simulink model "VSG_2level"  (R2024b)
settings: Solver=ode23t  StartTime=0.0  StopTime=4  RelTol=1e-3
InitFcn:
  | Rf = 0.05;
  | fn = 50;
  | Ub = 380;
  | Sb = 150e3;
  | Ib = Sb/(sqrt(3)*Ub);
  | W0 = 2*pi*fn;
  | J = 3.36;
  | D = 3.24e4/W0;
  | Kf = 2.941e6/W0;
  | Kq = (9e4*Ub)/(Sb*sqrt(3));
  | Ki = 0.35*sqrt(3)*Sb/Ub;
  | L = 1e-3;
  | Cf = 35e-6;
  | R = 0.1;
  | Un = 380;
undefined symbols (not defined in the file or in its folder): Ion, Lithium
libraries: spsSeriesRLCBranchLib x13, spsIGBTDiodeLib x10, slpidlib x7, spsThreePhaseVIMeasurementLib x4, spsabctodq0Lib x4, spsVoltageMeasurementLib x4, spsPowerPositiveSequenceLib x3, simulink x3, spsBatteryLib x2, spsPLL3phLib x2, spsThreePhaseSeriesRLCLoadLib x2, spsThreePhaseBreakerLib x2
(part 1 of 2)
settings Model: Creator=ASUS  LastModifiedBy=ASUS
settings DataIOCC: ReturnWorkspaceOutputs=off

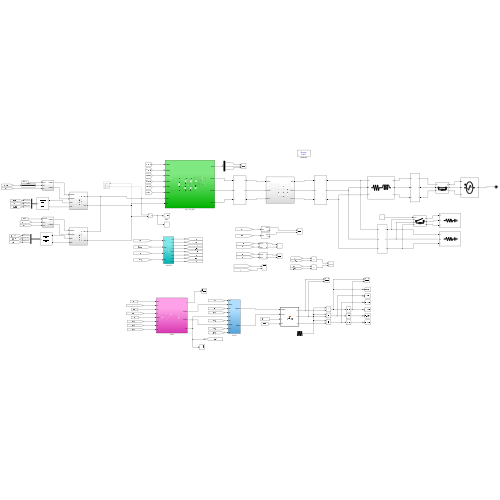
[thumbnail: Simulink's stored preview of the top-level diagram]
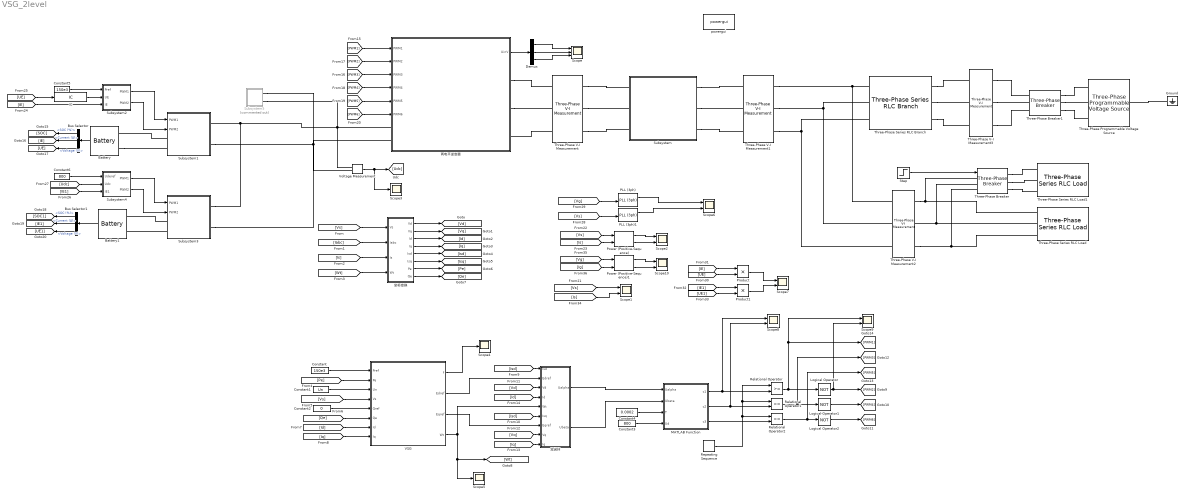
== system VSG_2level ==
  Battery : spsBatteryLib/Battery  BatType=Lithium-Ion  NomV=500  NomQ=100  SOC=80  Batt_Tr=30  PresetModel=on  MaxQ=100  MinV=375  FullV=581.9936  Dis_rate=43.4783  R=0.05  Normal_OP=90.4348  expZone="[540.1929      4.913043]"
  Battery1 : spsBatteryLib/Battery  BatType=Lithium-Ion  NomV=500  NomQ=50  SOC=80  Batt_Tr=30  PresetModel=on  MaxQ=50  MinV=375  FullV=581.9936  Dis_rate=21.7391  R=0.1  Normal_OP=45.2174  expZone="[540.1929      2.456522]"
  Bus Selector : BusSelector  OutputSignals=SOC (%),Current (A),Voltage (V)
  Bus Selector1 : BusSelector  OutputSignals=SOC (%),Current (A),Voltage (V)
  Constant : Constant  Value=150e3
  Constant1 : Constant  Value=Un
  Constant2 : Constant  Value=0
  Constant3 : Constant  Value=800
  Constant4 : Constant  Value=0.0002
  Constant5 : Constant  Value=150e3
  Constant6 : Constant  Value=800
  Demux : Demux  Outputs=3
  Ground : spsGroundLib/Ground  LConnTagsString=a
  IC : InitialCondition  Value=800
  Logical Operator : Logic  Operator=NOT  AllPortsSameDT=off  OutDataTypeStr=boolean
  Logical Operator1 : Logic  Operator=NOT  AllPortsSameDT=off  OutDataTypeStr=boolean
  Logical Operator2 : Logic  Operator=NOT  AllPortsSameDT=off  OutDataTypeStr=boolean
  MATLAB Function : MATLAB Function  TreatAsAtomicUnit=on
  PLL (3ph) : spsPLL3phLib/PLL (3ph)  Fmin=45  Par_Init=[0, 50]  ParK=[180, 3200, 1]  TcD=1e-4  MaxRateChangeFreq=12  FilterCutOffFreq=25  Ts=0  AGC=on
  PLL (3ph)1 : spsPLL3phLib/PLL (3ph)  Fmin=45  Par_Init=[0, 50]  ParK=[180, 3200, 1]  TcD=1e-4  MaxRateChangeFreq=12  FilterCutOffFreq=25  Ts=0  AGC=on
  Power (Positive-Sequence) : spsPowerPositiveSequenceLib/Power (Positive-Sequence)  Freq=60  Vinit=[0, 0]  Iinit=[0, 0]  Ts=0
      settings: LibrarySourceBlock=|
      | sps_lib/Sensors and Measurements/Power
      | (Positive-Sequence)
  Power (Positive-Sequence)1 : spsPowerPositiveSequenceLib/Power (Positive-Sequence)  Freq=60  Vinit=[0, 0]  Iinit=[0, 0]  Ts=0
      settings: LibrarySourceBlock=|
      | sps_lib/Sensors and Measurements/Power
      | (Positive-Sequence)
  Product : Product
  Product1 : Product
  Relational Operator : RelationalOperator  OutDataTypeStr=boolean  RndMeth=Simplest  InputSameDT=off
  Relational Operator1 : RelationalOperator  OutDataTypeStr=boolean  RndMeth=Simplest  InputSameDT=off
  Relational Operator2 : RelationalOperator  OutDataTypeStr=boolean  RndMeth=Simplest  InputSameDT=off
  Repeating Sequence : simulink/Sources/Repeating Sequence  rep_seq_t=[0 1/10000 0.0002]  rep_seq_y=[0 1/10000 0]
  Scope : Scope  NumInputPorts=3
  Scope{1..2,6..10} (7 alike) : Scope  NumInputPorts=2
  Scope3 : Scope
  Scope4 : Scope
  Scope5 : Scope
  Step : Step  SampleTime=0
  Subsystem : Subsystem
  Subsystem1 : Subsystem
  Subsystem2 : Subsystem
  Subsystem3 : Subsystem
  Subsystem4 : Subsystem
  Subsystem5 : Subsystem  Commented=on
  Three-Phase Programmable Voltage Source : spsThreePhaseProgrammableVoltageSourceLib/Three-Phase Programmable Voltage Source  PositiveSequence=[380 0 50]  VariationEntity=Frequency  VariationType=Table of time-amplitude pairs  VariationTypeAlt=Step  VariationStep=0  VariationRate=10  VariationMagnitude=0.3  VariationFrequency=2  VariationTiming=[0 0]  VariationPhaseA=off  Amplitudes=[1 0.8 1.2 1.0]  TimeValues=[0 0.1 0.15 0.2]  HarmonicGeneration=off  HarmonicA=[3 0.2 -25 0]  HarmonicB=[2 0.15 35 2]  Timing="[0.05  3]"  BusType=swing  Pref=0  Qref=0  Qmin=-inf  Qmax=inf
  Three-Phase Series RLC Branch : spsThreePhaseSeriesRLCBranchLib/Three-Phase Series RLC Branch  LConnTagsString=A|B|C  RConnTagsString=A|B|C  BranchType=RL  Resistance=0.06  Inductance=1.35e-3  Capacitance=1e-6  Measurements=None
  Three-Phase Series RLC Load : spsThreePhaseSeriesRLCLoadLib/Three-Phase Series RLC Load  LConnTagsString=A|B|C  Configuration=Y (grounded)  NominalVoltage=380  Vabc=[1e3 1e3 1e3]  Vabcp=[1e3 1e3 1e3]  NominalFrequency=50  UnbalancedPower=off  ActivePower=100e3  InductivePower=0  CapacitivePower=0  Pabc=[10e3 9e3 11e3]  QLabc=[100 90 110]  QCabc=[100 90 110]  Pabcp=[10e3 9e3 11e3]  QLabcp=[100 90 110]  QCabcp=[100 90 110]  Measurements=None  LoadType=constant Z
  Three-Phase Series RLC Load1 : spsThreePhaseSeriesRLCLoadLib/Three-Phase Series RLC Load  LConnTagsString=A|B|C  Configuration=Y (grounded)  NominalVoltage=380  Vabc=[1e3 1e3 1e3]  Vabcp=[1e3 1e3 1e3]  NominalFrequency=50  UnbalancedPower=off  ActivePower=50e3  InductivePower=0  CapacitivePower=0  Pabc=[10e3 9e3 11e3]  QLabc=[100 90 110]  QCabc=[100 90 110]  Pabcp=[10e3 9e3 11e3]  QLabcp=[100 90 110]  QCabcp=[100 90 110]  Measurements=None  LoadType=constant Z
  Three-Phase V-I Measurement : spsThreePhaseVIMeasurementLib/Three-Phase V-I Measurement  VoltageMeasurement=no  SetLabelV=off  LabelV=Vabc  Vpu=off  VpuLL=off  CurrentMeasurement=yes  SetLabelI=on  LabelI=Iabc  Ipu=off  Pbase=100e6  Vbase=500e3  OutputType=Complex  PhasorSimulation=off  PSBequivalent=0
  Three-Phase V-I Measurement1 : spsThreePhaseVIMeasurementLib/Three-Phase V-I Measurement  VoltageMeasurement=phase-to-ground  SetLabelV=on  LabelV=Vs  Vpu=off  VpuLL=off  CurrentMeasurement=yes  SetLabelI=on  LabelI=Is  Ipu=off  Pbase=100e6  Vbase=500e3  OutputType=Complex  PhasorSimulation=off  PSBequivalent=0
  Three-Phase V-I Measurement2 : spsThreePhaseVIMeasurementLib/Three-Phase V-I Measurement  VoltageMeasurement=phase-to-ground  SetLabelV=on  LabelV=VL  Vpu=off  VpuLL=off  CurrentMeasurement=yes  SetLabelI=on  LabelI=IL  Ipu=off  Pbase=100e6  Vbase=500e3  OutputType=Complex  PhasorSimulation=off  PSBequivalent=0
  Three-Phase V-I Measurement3 : spsThreePhaseVIMeasurementLib/Three-Phase V-I Measurement  VoltageMeasurement=phase-to-ground  SetLabelV=on  LabelV=Vg  Vpu=off  VpuLL=off  CurrentMeasurement=yes  SetLabelI=on  LabelI=Ig  Ipu=off  Pbase=100e6  Vbase=500e3  OutputType=Complex  PhasorSimulation=off  PSBequivalent=0
  Three-Phase Breaker : spsThreePhaseBreakerLib/Three-Phase Breaker  InitialState=open  SwitchA=on  SwitchB=on  SwitchC=on  SwitchTimes="[1  5/60]"  External=on  BreakerResistance=0.0000001  SnubberResistance=1e10  SnubberCapacitance=inf  Measurements=None
  Three-Phase Breaker1 : spsThreePhaseBreakerLib/Three-Phase Breaker  InitialState=closed  SwitchA=on  SwitchB=on  SwitchC=on  SwitchTimes=[2]  External=off  BreakerResistance=0.0000001  SnubberResistance=1e10  SnubberCapacitance=inf  Measurements=None
  VSG : Subsystem
  Voltage Measurement : spsVoltageMeasurementLib/Voltage Measurement  PhasorSimulation=off  OutputType=Complex  PSBequivalent=0
  powergui : sps_lib/powergui  Priority=1  SimulationMode=Discrete  SampleTime=1e-6  frequency=60  Iterations=50  frequencyindice=0  Pbase=100e6  ErrMax=1e-4  UnitsV=kV  UnitsW=MW  buscounter=0  FunctionMessages=off  echomessages=off  EnableUseOfTLC=off  CurrentSourceSwitches=off  DisableSnubberDevices=off  DisableRonSwitches=off  DisableVfSwitches=off  DisplayEquations=off  AutomaticDiscreteSolvers=off  SolverType=Tustin/Backward Euler (TBE)  Interpol=off  ExternalGateDelay=off  methode=off  Ts=100  x0status=blocks  SPID=on  SwTol=0  HookPort=off  NonlinearTolerance=1e-4  nMaxIteration=100  ContinueOnMaxIteration=off  RestoreLinks=warning  ResistiveCurrentMeasurement=off  Frange=[0:2:500]  Ylog=off  Xlog=on  ShowGrid=off  save=off  variable=ZData  structure=0  ZoomFFT=off  StartTime=0.0  cycles=1  DisplayStyle=1  fundamental=60  FreqAxis=off  MaxFrequency=1000  frequencyindicesteady=1  RmsSteady=1  display=off
  两电平逆变器 : Subsystem
  双闭环 : Subsystem
  坐标变换 : Subsystem
  wires:
  [Vs] -> 坐标变换/1(Vs)
  [Iabc] -> 坐标变换/2(Iabc)
  [Is] -> 坐标变换/3(Is)
  [Wt] -> 坐标变换/4(Wt)
  坐标变换/1(Vd) -> [Vd]
  坐标变换/2(Vq) -> [Vq]
  坐标变换/3(Id) -> [Id]
  坐标变换/4(Iq) -> [Iq]
  坐标变换/5(Isd) -> [Isd]
  坐标变换/6(Isq) -> [Isq]
  坐标变换/7(Pe) -> [Pe]
  坐标变换/8(Qe) -> [Qe]
  Constant/1 -> VSG/1(Pref)
  [Pe] -> VSG/2(Pe)
  Constant1/1 -> VSG/3(Un)
  [Vs] -> VSG/4(Vs)
  Constant2/1 -> VSG/5(Qref)
  [Qe] -> VSG/6(Qe)
  [Id] -> VSG/7(Id)
  [Iq] -> VSG/8(Iq)
  VSG/2(Edref) -> 双闭环/2(Edref)
  VSG/3(Eqref) -> 双闭环/7(Eqref)
  [Isd] -> 双闭环/1(Isd)
  [Isd] -> 双闭环/6(Isq)
  VSG/4(Wt) -> 双闭环/5(Wt), [Wt], Scope5/1
  [Vd] -> 双闭环/3(Vd)
  [Vq] -> 双闭环/8(Vq)
  [Iq] -> 双闭环/9(Iq)
  [Id] -> 双闭环/4(Id)
  双闭环/1(Ualpha) -> MATLAB Function/1(Ualpha)
  双闭环/2(Ubeta) -> MATLAB Function/2(Ubeta)
  Constant3/1 -> MATLAB Function/4(Ud)
  Constant4/1 -> MATLAB Function/3(T)
  Repeating Sequence/1 -> Relational Operator2/1, Relational Operator1/1, Relational Operator/1
  MATLAB Function/1(c1) -> Scope8/1, Relational Operator/2
  MATLAB Function/2(c2) -> Scope8/2, Relational Operator1/2
  MATLAB Function/3(c3) -> Relational Operator2/2
  Relational Operator/1 -> Scope9/1, [PWM1], Logical Operator/1
  Relational Operator1/1 -> [PWM3], Logical Operator1/1
  Relational Operator2/1 -> [PWM5], Logical Operator2/1
  Logical Operator/1 -> Scope9/2, [PWM2]
  Logical Operator1/1 -> [PWM4]
  Logical Operator2/1 -> [PWM6]
  [PWM6] -> 两电平逆变器/6(PWM6)
  [PWM5] -> 两电平逆变器/5(PWM5)
  [PWM4] -> 两电平逆变器/4(PWM4)
  [PWM3] -> 两电平逆变器/3(PWM3)
  [PWM2] -> 两电平逆变器/2(PWM2)
  [PWM1] -> 两电平逆变器/1(PWM1)
  两电平逆变器/1(UinV) -> Demux/1
  Demux/2 -> Scope/2
  Demux/1 -> Scope/1
  Demux/3 -> Scope/3
  [Vs] -> Scope1/1
  [Vs] -> Power (Positive-Sequence)/1
  [Is] -> Power (Positive-Sequence)/2
  Power (Positive-Sequence)/1 -> Scope2/1
  Power (Positive-Sequence)/2 -> Scope2/2
  Battery/1 -> Bus Selector/1
  Bus Selector/1 -> [SOC]  "<SOC (%)>"
  Bus Selector/2 -> [IE]  "<Current (A)>"
  Bus Selector/3 -> [UE]  "<Voltage (V)>"
  [UE] -> IC/1
  [IE] -> Subsystem2/3(IE)
  Constant5/1 -> Subsystem2/1(Pref)
  Subsystem2/1(PWM1) -> Subsystem1/1(PWM1)
  Subsystem2/2(PWM2) -> Subsystem1/2(PWM2)
  Subsystem4/2(PWM2) -> Subsystem3/2(PWM2)
  Subsystem4/1(PWM1) -> Subsystem3/1(PWM1)
  Constant6/1 -> Subsystem4/1(Uderef)
  [IE1] -> Subsystem4/3(IE1)
  [Udc] -> Subsystem4/2(Udc)
  Bus Selector1/3 -> [UE1]  "<Voltage (V)>"
  Bus Selector1/2 -> [IE1]  "<Current (A)>"
  Bus Selector1/1 -> [SOC1]  "<SOC (%)>"
  Battery1/1 -> Bus Selector1/1
  Voltage Measurement/1 -> Scope3/1, [Udc]
  IC/1 -> Subsystem2/2(UE)
  VSG/1(f) -> Scope4/1
  [Vg] -> PLL (3ph)/1
  [Vs] -> PLL (3ph)1/1
  PLL (3ph)/1 -> Scope6/1
  PLL (3ph)1/1 -> Scope6/2
  [IE] -> Product/1
  [UE] -> Product/2
  [UE1] -> Product1/2
  [IE1] -> Product1/1
  Product/1 -> Scope7/1
  Product1/1 -> Scope7/2
  [Is] -> Scope1/2
  Power (Positive-Sequence)1/2 -> Scope10/2
  Power (Positive-Sequence)1/1 -> Scope10/1
  [Ig] -> Power (Positive-Sequence)1/2
  [Vg] -> Power (Positive-Sequence)1/1
  Step/1 -> Three-Phase Breaker/1
  connections:
  两电平逆变器/RConn1 -- Three-Phase V-I Measurement/LConn1
  两电平逆变器/RConn2 -- Three-Phase V-I Measurement/LConn2
  Three-Phase V-I Measurement/LConn3 -- 两电平逆变器/RConn3
  Three-Phase V-I Measurement/RConn1 -- Subsystem/LConn1
  Three-Phase V-I Measurement/RConn2 -- Subsystem/LConn2
  Three-Phase V-I Measurement/RConn3 -- Subsystem/LConn3
  Subsystem/RConn1 -- Three-Phase V-I Measurement1/LConn1
  Subsystem/RConn2 -- Three-Phase V-I Measurement1/LConn2
  Subsystem/RConn3 -- Three-Phase V-I Measurement1/LConn3
  Three-Phase V-I Measurement2/RConn1 -- Three-Phase Breaker/LConn1 -- Three-Phase Series RLC Load/LConn1
  Three-Phase Series RLC Load/LConn2 -- Three-Phase Breaker/LConn2 -- Three-Phase V-I Measurement2/RConn2
  Three-Phase V-I Measurement2/RConn3 -- Three-Phase Breaker/LConn3 -- Three-Phase Series RLC Load/LConn3
  Three-Phase V-I Measurement1/RConn1 -- Three-Phase Series RLC Branch/LConn1 -- Three-Phase V-I Measurement2/LConn1
  Three-Phase V-I Measurement1/RConn2 -- Three-Phase Series RLC Branch/LConn2 -- Three-Phase V-I Measurement2/LConn2
  Three-Phase V-I Measurement1/RConn3 -- Three-Phase Series RLC Branch/LConn3 -- Three-Phase V-I Measurement2/LConn3
  Three-Phase Series RLC Branch/RConn1 -- Three-Phase V-I Measurement3/LConn1
  Three-Phase Series RLC Branch/RConn2 -- Three-Phase V-I Measurement3/LConn2
  Three-Phase Series RLC Branch/RConn3 -- Three-Phase V-I Measurement3/LConn3
  Ground/LConn1 -- Three-Phase Programmable Voltage Source/LConn1
  Battery/LConn2 -- Subsystem1/LConn2
  Subsystem3/LConn2 -- Battery1/LConn2
  Subsystem3/LConn1 -- Battery1/LConn1
  两电平逆变器/LConn1 -- Subsystem3/RConn1 -- Subsystem1/RConn1 -- Subsystem5/LConn2 -- Voltage Measurement/LConn1
  Subsystem1/RConn2 -- Subsystem5/LConn1 -- 两电平逆变器/LConn2 -- Subsystem3/RConn2 -- Voltage Measurement/LConn2
  Subsystem1/LConn1 -- Battery/LConn1
  Three-Phase Breaker/RConn2 -- Three-Phase Series RLC Load1/LConn2
  Three-Phase Breaker/RConn3 -- Three-Phase Series RLC Load1/LConn3
  Three-Phase V-I Measurement3/RConn1 -- Three-Phase Breaker1/LConn1
  Three-Phase V-I Measurement3/RConn2 -- Three-Phase Breaker1/LConn2
  Three-Phase V-I Measurement3/RConn3 -- Three-Phase Breaker1/LConn3
  Three-Phase Breaker1/RConn2 -- Three-Phase Programmable Voltage Source/RConn2
  Three-Phase Breaker1/RConn1 -- Three-Phase Programmable Voltage Source/RConn1
  Three-Phase Breaker1/RConn3 -- Three-Phase Programmable Voltage Source/RConn3
  Three-Phase Breaker/RConn1 -- Three-Phase Series RLC Load1/LConn1

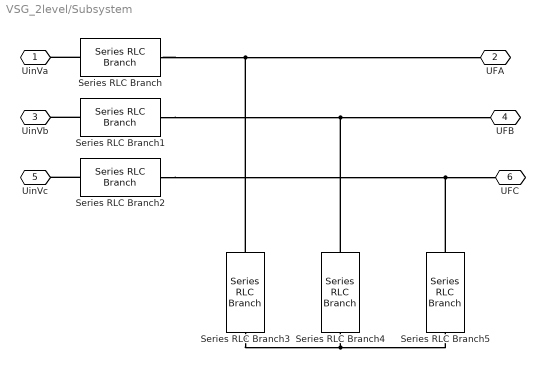
== system VSG_2level/Subsystem ==
  Series RLC Branch : spsSeriesRLCBranchLib/Series RLC Branch  LConnTagsString=__new0  RConnTagsString=__new0  BranchType=RL  Resistance=Rf  Inductance=L  SetiL0=off  InitialCurrent=0  Capacitance=1e-6  Setx0=off  InitialVoltage=0  Measurements=None
  Series RLC Branch1 : spsSeriesRLCBranchLib/Series RLC Branch  LConnTagsString=__new0  RConnTagsString=__new0  BranchType=RL  Resistance=Rf  Inductance=L  SetiL0=off  InitialCurrent=0  Capacitance=1e-6  Setx0=off  InitialVoltage=0  Measurements=None
  Series RLC Branch2 : spsSeriesRLCBranchLib/Series RLC Branch  LConnTagsString=__new0  RConnTagsString=__new0  BranchType=RL  Resistance=Rf  Inductance=L  SetiL0=off  InitialCurrent=0  Capacitance=1e-6  Setx0=off  InitialVoltage=0  Measurements=None
  Series RLC Branch3 : spsSeriesRLCBranchLib/Series RLC Branch  LConnTagsString=__new0  RConnTagsString=__new0  BranchType=RC  Resistance=Rf  Inductance=L  SetiL0=off  InitialCurrent=0  Capacitance=Cf  Setx0=off  InitialVoltage=0  Measurements=None
  Series RLC Branch4 : spsSeriesRLCBranchLib/Series RLC Branch  LConnTagsString=__new0  RConnTagsString=__new0  BranchType=RC  Resistance=Rf  Inductance=L  SetiL0=off  InitialCurrent=0  Capacitance=Cf  Setx0=off  InitialVoltage=0  Measurements=None
  Series RLC Branch5 : spsSeriesRLCBranchLib/Series RLC Branch  LConnTagsString=__new0  RConnTagsString=__new0  BranchType=RC  Resistance=Rf  Inductance=L  SetiL0=off  InitialCurrent=0  Capacitance=Cf  Setx0=off  InitialVoltage=0  Measurements=None
  UinVa : PMIOPort  Side=Left
  UFA : PMIOPort  Port=2  Side=Right
  UinVb : PMIOPort  Port=3  Side=Left
  UFB : PMIOPort  Port=4  Side=Right
  UinVc : PMIOPort  Port=5  Side=Left
  UFC : PMIOPort  Port=6  Side=Right
  connections:
  Series RLC Branch3/RConn1 -- Series RLC Branch5/RConn1 -- Series RLC Branch4/RConn1
  Series RLC Branch/RConn1 -- UFA/RConn1 -- Series RLC Branch3/LConn1
  Series RLC Branch2/RConn1 -- UFC/RConn1 -- Series RLC Branch5/LConn1
  Series RLC Branch1/RConn1 -- UFB/RConn1 -- Series RLC Branch4/LConn1
  Series RLC Branch1/LConn1 -- UinVb/RConn1
  Series RLC Branch/LConn1 -- UinVa/RConn1
  Series RLC Branch2/LConn1 -- UinVc/RConn1

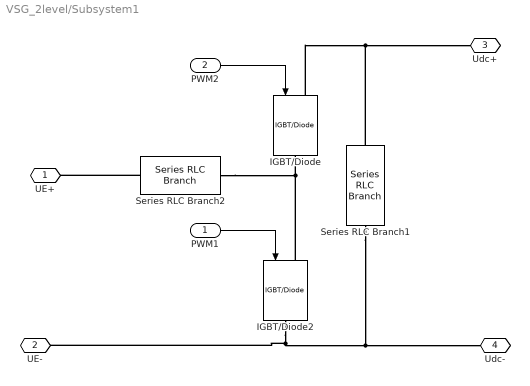
== system VSG_2level/Subsystem1 ==
  PWM1 : Inport
  PWM2 : Inport  Port=2
  IGBT/Diode : spsIGBTDiodeLib/IGBT//Diode  Ron=1e-3  Rs=1e5  Cs=inf  Measurements=off
  IGBT/Diode2 : spsIGBTDiodeLib/IGBT//Diode  Ron=1e-3  Rs=1e5  Cs=inf  Measurements=off
  Series RLC Branch1 : spsSeriesRLCBranchLib/Series RLC Branch  LConnTagsString=__new0  RConnTagsString=__new0  BranchType=C  Resistance=1  Inductance=1.68e-3  SetiL0=off  InitialCurrent=0  Capacitance=5.5e-3  Setx0=on  InitialVoltage=800  Measurements=None
  Series RLC Branch2 : spsSeriesRLCBranchLib/Series RLC Branch  LConnTagsString=__new0  RConnTagsString=__new0  BranchType=L  Resistance=1  Inductance=1.68e-3  SetiL0=off  InitialCurrent=0  Capacitance=1e-6  Setx0=off  InitialVoltage=0  Measurements=None
  UE+ : PMIOPort  Side=Left
  UE- : PMIOPort  Port=2  Side=Left
  Udc+ : PMIOPort  Port=3  Side=Right
  Udc- : PMIOPort  Port=4  Side=Right
  wires:
  PWM1/1 -> IGBT/Diode2/1
  PWM2/1 -> IGBT/Diode/1
  connections:
  Series RLC Branch2/LConn1 -- UE+/RConn1
  IGBT/Diode2/LConn1 -- IGBT/Diode/RConn1 -- Series RLC Branch2/RConn1
  IGBT/Diode/LConn1 -- Udc+/RConn1 -- Series RLC Branch1/LConn1
  IGBT/Diode2/RConn1 -- UE-/RConn1 -- Udc-/RConn1 -- Series RLC Branch1/RConn1

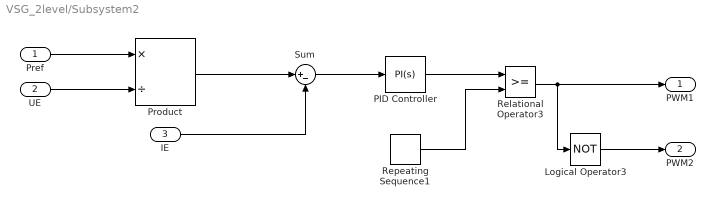
== system VSG_2level/Subsystem2 ==
  Pref : Inport
  UE : Inport  Port=2
  IE : Inport  Port=3
  Logical Operator3 : Logic  Operator=NOT  AllPortsSameDT=off  OutDataTypeStr=boolean
  PID Controller : slpidlib/PID Controller  Controller=PI  Form=Parallel  TimeDomain=Continuous-time  UseExternalTs=off  SampleTime=-1  IntegratorMethod=Forward Euler  FilterMethod=Forward Euler  ControllerParametersSource=internal  P=0.715  I=1.12  UseKiTs=off  D=0  UseExternalDerivativeSource=off  N=100  UseFilter=on  TunerSelectOption=Transfer Function Based (PID Tuner App)  InitialConditionSource=internal  InitialConditionForIntegrator=0  InitialConditionForFilter=0  DifferentiatorICPrevScaledInput=0  ExternalReset=none  TrackingMode=off  Kt=1  LimitOutput=off  SatLimitsSource=internal  UpperSaturationLimit=1e10  LowerSaturationLimit=-1e10  LinearizeAsGain=on  AntiWindupMode=none  Kb=1  LimitIntegrator=off  UpperIntegratorSaturationLimit=1e10  LowerIntegratorSaturationLimit=-1e10  POutMin=[]  POutMax=[]  IOutMin=[]  IOutMax=[]  DOutMin=[]  DOutMax=[]  NOutMin=[]  NOutMax=[]  SumOutMin=[]  SumOutMax=[]  SaturationOutMin=[]  SaturationOutMax=[]  PParamMin=[]  PParamMax=[]  IParamMin=[]  IParamMax=[]  DParamMin=[]  DParamMax=[]  NParamMin=[]  NParamMax=[]  KbParamMin=[]  KbParamMax=[]  KtParamMin=[]  KtParamMax=[]  KbOutMin=[]  KbOutMax=[]  KtOutMin=[]  KtOutMax=[]  IntegratorOutMin=[]  IntegratorOutMax=[]  FilterOutMin=[]  FilterOutMax=[]  SumI1OutMin=[]  SumI1OutMax=[]  SumI2OutMin=[]  SumI2OutMax=[]  SumI3OutMin=[]  SumI3OutMax=[]  SumI4OutMin=[]  SumI4OutMax=[]  SumDOutMin=[]  SumDOutMax=[]  DifferentiatorOutMin=[]  DifferentiatorOutMax=[]  FilterDiffOutCoefMin=[]  FilterDiffOutCoefMax=[]  ReciprocalOutMin=[]  ReciprocalOutMax=[]  SumDenOutMin=[]  SumDenOutMax=[]  SumNumOutMin=[]  SumNumOutMax=[]  DivideOutMin=[]  DivideOutMax=[]  UdiffTsProdOutMin=[]  UdiffTsProdOutMax=[]  NTsProdOutMin=[]  NTsProdOutMax=[]  UintegralTsProdOutMin=[]  UintegralTsProdOutMax=[]  UngainTsProdOutMin=[]  UngainTsProdOutMax=[]  ClampingZeroOutDataTypeStr=Inherit: Inherit via back propagation  ClampingZeroOutMin=[]  ClampingZeroOutMax=[]  FilterDenConstantOutDataTypeStr=Inherit: Inherit via back propagation  FilterDenConstantOutMin=[]  FilterDenConstantOutMax=[]  PCopyOutDataTypeStr=Inherit: Inherit via back propagation  PCopyOutMin=[]  PCopyOutMax=[]  NCopyOutDataTypeStr=Inherit: Inherit via back propagation  NCopyOutMin=[]  NCopyOutMax=[]  IntegratorContinuousStateAttributes=''  IntegratorStateMustResolveToSignalObject=off  IntegratorRTWStateStorageClass=Auto  FilterContinuousStateAttributes=''  FilterStateMustResolveToSignalObject=off  FilterRTWStateStorageClass=Auto  ParallelPVariant=InternalParameters  IdealPVariant=Disabled  IVariant=InternalParameters  DVariant=Disabled  IntegratorVariant=Continuous  SatVariant=Disabled  AWVariant=Passthrough  PCopyVariant=Disabled  TRVariant=Disabled  FdbkBlocksVariant=Forward  IdealPFdbkVariant=Disabled  SatFdbkVariant=Disabled  DerivativeFilterVariant=Disabled  NVariant=Disabled  NCopyVariant=Disabled_SignalSpec  FilterICVariant=Disabled  IntegratorICVariant=InternalICs  ExternalResetVariant=Disabled  TRSumVariant=Passthrough  SumFdbkVariant=Disabled  SumVariant=Sum_PI  TsampFilterVariant=InternalTs  TsampNgainVariant=Passthrough  TsampIntegralVariant=Disabled_SignalSpec  ExternalSaturationOutDataTypeStr=Inherit: Same as second input  DerivativeSourceVariant=Disabled  PreIntVariant=InternalPreInt
  Product : Product  Inputs=*/
  Relational Operator3 : RelationalOperator  OutDataTypeStr=boolean  RndMeth=Simplest  InputSameDT=off
  Repeating Sequence1 : simulink/Sources/Repeating Sequence  rep_seq_t=[0 0.0001]  rep_seq_y=[0 1]
  Sum : Sum  Inputs=|+-
  PWM1 : Outport
  PWM2 : Outport  Port=2
  wires:
  Sum/1 -> PID Controller/1
  Product/1 -> Sum/1
  Pref/1 -> Product/1
  UE/1 -> Product/2
  IE/1 -> Sum/2
  Logical Operator3/1 -> PWM2/1
  Relational Operator3/1 -> PWM1/1, Logical Operator3/1
  Repeating Sequence1/1 -> Relational Operator3/2
  PID Controller/1 -> Relational Operator3/1

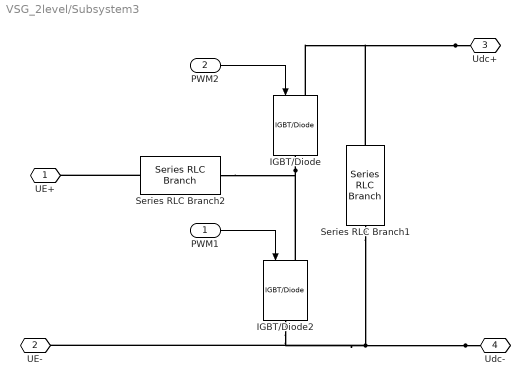
== system VSG_2level/Subsystem3 ==
  PWM1 : Inport
  PWM2 : Inport  Port=2
  IGBT/Diode : spsIGBTDiodeLib/IGBT//Diode  Ron=1e-3  Rs=1e5  Cs=inf  Measurements=off
  IGBT/Diode2 : spsIGBTDiodeLib/IGBT//Diode  Ron=1e-3  Rs=1e5  Cs=inf  Measurements=off
  Series RLC Branch1 : spsSeriesRLCBranchLib/Series RLC Branch  LConnTagsString=__new0  RConnTagsString=__new0  BranchType=C  Resistance=1  Inductance=1.68e-3  SetiL0=off  InitialCurrent=0  Capacitance=5.5e-3  Setx0=on  InitialVoltage=800  Measurements=None
  Series RLC Branch2 : spsSeriesRLCBranchLib/Series RLC Branch  LConnTagsString=__new0  RConnTagsString=__new0  BranchType=L  Resistance=1  Inductance=1.68e-3  SetiL0=off  InitialCurrent=0  Capacitance=1e-6  Setx0=off  InitialVoltage=0  Measurements=None
  UE+ : PMIOPort  Side=Left
  UE- : PMIOPort  Port=2  Side=Left
  Udc+ : PMIOPort  Port=3  Side=Right
  Udc- : PMIOPort  Port=4  Side=Right
  wires:
  PWM2/1 -> IGBT/Diode/1
  PWM1/1 -> IGBT/Diode2/1
  connections:
  Udc-/RConn1 -- IGBT/Diode2/RConn1 -- UE-/RConn1 -- Series RLC Branch1/RConn1
  Udc+/RConn1 -- IGBT/Diode/LConn1 -- Series RLC Branch1/LConn1
  IGBT/Diode/RConn1 -- Series RLC Branch2/RConn1 -- IGBT/Diode2/LConn1
  Series RLC Branch2/LConn1 -- UE+/RConn1

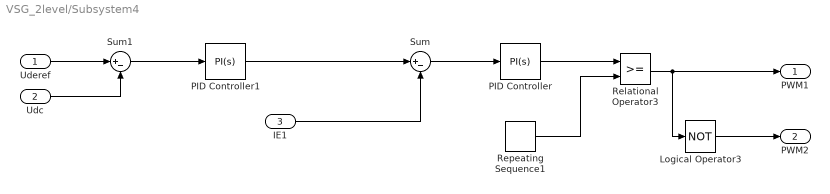
== system VSG_2level/Subsystem4 ==
  Uderef : Inport
  Udc : Inport  Port=2
  IE1 : Inport  Port=3
  Logical Operator3 : Logic  Operator=NOT  AllPortsSameDT=off  OutDataTypeStr=boolean
  PID Controller : slpidlib/PID Controller  Controller=PI  Form=Parallel  TimeDomain=Continuous-time  UseExternalTs=off  SampleTime=-1  IntegratorMethod=Forward Euler  FilterMethod=Forward Euler  ControllerParametersSource=internal  P=2.75  I=3.12  UseKiTs=off  D=0  UseExternalDerivativeSource=off  N=100  UseFilter=on  TunerSelectOption=Transfer Function Based (PID Tuner App)  InitialConditionSource=internal  InitialConditionForIntegrator=0  InitialConditionForFilter=0  DifferentiatorICPrevScaledInput=0  ExternalReset=none  TrackingMode=off  Kt=1  LimitOutput=off  SatLimitsSource=internal  UpperSaturationLimit=inf  LowerSaturationLimit=-inf  LinearizeAsGain=on  AntiWindupMode=none  Kb=1  LimitIntegrator=off  UpperIntegratorSaturationLimit=inf  LowerIntegratorSaturationLimit=-inf  POutMin=[]  POutMax=[]  IOutMin=[]  IOutMax=[]  DOutMin=[]  DOutMax=[]  NOutMin=[]  NOutMax=[]  SumOutMin=[]  SumOutMax=[]  SaturationOutMin=[]  SaturationOutMax=[]  PParamMin=[]  PParamMax=[]  IParamMin=[]  IParamMax=[]  DParamMin=[]  DParamMax=[]  NParamMin=[]  NParamMax=[]  KbParamMin=[]  KbParamMax=[]  KtParamMin=[]  KtParamMax=[]  KbOutMin=[]  KbOutMax=[]  KtOutMin=[]  KtOutMax=[]  IntegratorOutMin=[]  IntegratorOutMax=[]  FilterOutMin=[]  FilterOutMax=[]  SumI1OutMin=[]  SumI1OutMax=[]  SumI2OutMin=[]  SumI2OutMax=[]  SumI3OutMin=[]  SumI3OutMax=[]  SumI4OutMin=[]  SumI4OutMax=[]  SumDOutMin=[]  SumDOutMax=[]  DifferentiatorOutMin=[]  DifferentiatorOutMax=[]  FilterDiffOutCoefMin=[]  FilterDiffOutCoefMax=[]  ReciprocalOutMin=[]  ReciprocalOutMax=[]  SumDenOutMin=[]  SumDenOutMax=[]  SumNumOutMin=[]  SumNumOutMax=[]  DivideOutMin=[]  DivideOutMax=[]  UdiffTsProdOutMin=[]  UdiffTsProdOutMax=[]  NTsProdOutMin=[]  NTsProdOutMax=[]  UintegralTsProdOutMin=[]  UintegralTsProdOutMax=[]  UngainTsProdOutMin=[]  UngainTsProdOutMax=[]  ClampingZeroOutDataTypeStr=Inherit: Inherit via back propagation  ClampingZeroOutMin=[]  ClampingZeroOutMax=[]  FilterDenConstantOutDataTypeStr=Inherit: Inherit via back propagation  FilterDenConstantOutMin=[]  FilterDenConstantOutMax=[]  PCopyOutDataTypeStr=Inherit: Inherit via back propagation  PCopyOutMin=[]  PCopyOutMax=[]  NCopyOutDataTypeStr=Inherit: Inherit via back propagation  NCopyOutMin=[]  NCopyOutMax=[]  IntegratorContinuousStateAttributes=''  IntegratorStateMustResolveToSignalObject=off  IntegratorRTWStateStorageClass=Auto  FilterContinuousStateAttributes=''  FilterStateMustResolveToSignalObject=off  FilterRTWStateStorageClass=Auto  ParallelPVariant=InternalParameters  IdealPVariant=Disabled  IVariant=InternalParameters  DVariant=Disabled  IntegratorVariant=Continuous  SatVariant=Disabled  AWVariant=Passthrough  PCopyVariant=Disabled  TRVariant=Disabled  FdbkBlocksVariant=Forward  IdealPFdbkVariant=Disabled  SatFdbkVariant=Disabled  DerivativeFilterVariant=Disabled  NVariant=Disabled  NCopyVariant=Disabled_SignalSpec  FilterICVariant=Disabled  IntegratorICVariant=InternalICs  ExternalResetVariant=Disabled  TRSumVariant=Passthrough  SumFdbkVariant=Disabled  SumVariant=Sum_PI  TsampFilterVariant=InternalTs  TsampNgainVariant=Passthrough  TsampIntegralVariant=Disabled_SignalSpec  ExternalSaturationOutDataTypeStr=Inherit: Same as second input  DerivativeSourceVariant=Disabled  PreIntVariant=InternalPreInt
  PID Controller1 : slpidlib/PID Controller  Controller=PI  Form=Parallel  TimeDomain=Continuous-time  UseExternalTs=off  SampleTime=-1  IntegratorMethod=Forward Euler  FilterMethod=Forward Euler  ControllerParametersSource=internal  P=25  I=10.12  UseKiTs=off  D=0  UseExternalDerivativeSource=off  N=100  UseFilter=on  TunerSelectOption=Transfer Function Based (PID Tuner App)  InitialConditionSource=internal  InitialConditionForIntegrator=0  InitialConditionForFilter=0  DifferentiatorICPrevScaledInput=0  ExternalReset=none  TrackingMode=off  Kt=1  LimitOutput=off  SatLimitsSource=internal  UpperSaturationLimit=inf  LowerSaturationLimit=-inf  LinearizeAsGain=on  AntiWindupMode=none  Kb=1  LimitIntegrator=off  UpperIntegratorSaturationLimit=inf  LowerIntegratorSaturationLimit=-inf  POutMin=[]  POutMax=[]  IOutMin=[]  IOutMax=[]  DOutMin=[]  DOutMax=[]  NOutMin=[]  NOutMax=[]  SumOutMin=[]  SumOutMax=[]  SaturationOutMin=[]  SaturationOutMax=[]  PParamMin=[]  PParamMax=[]  IParamMin=[]  IParamMax=[]  DParamMin=[]  DParamMax=[]  NParamMin=[]  NParamMax=[]  KbParamMin=[]  KbParamMax=[]  KtParamMin=[]  KtParamMax=[]  KbOutMin=[]  KbOutMax=[]  KtOutMin=[]  KtOutMax=[]  IntegratorOutMin=[]  IntegratorOutMax=[]  FilterOutMin=[]  FilterOutMax=[]  SumI1OutMin=[]  SumI1OutMax=[]  SumI2OutMin=[]  SumI2OutMax=[]  SumI3OutMin=[]  SumI3OutMax=[]  SumI4OutMin=[]  SumI4OutMax=[]  SumDOutMin=[]  SumDOutMax=[]  DifferentiatorOutMin=[]  DifferentiatorOutMax=[]  FilterDiffOutCoefMin=[]  FilterDiffOutCoefMax=[]  ReciprocalOutMin=[]  ReciprocalOutMax=[]  SumDenOutMin=[]  SumDenOutMax=[]  SumNumOutMin=[]  SumNumOutMax=[]  DivideOutMin=[]  DivideOutMax=[]  UdiffTsProdOutMin=[]  UdiffTsProdOutMax=[]  NTsProdOutMin=[]  NTsProdOutMax=[]  UintegralTsProdOutMin=[]  UintegralTsProdOutMax=[]  UngainTsProdOutMin=[]  UngainTsProdOutMax=[]  ClampingZeroOutDataTypeStr=Inherit: Inherit via back propagation  ClampingZeroOutMin=[]  ClampingZeroOutMax=[]  FilterDenConstantOutDataTypeStr=Inherit: Inherit via back propagation  FilterDenConstantOutMin=[]  FilterDenConstantOutMax=[]  PCopyOutDataTypeStr=Inherit: Inherit via back propagation  PCopyOutMin=[]  PCopyOutMax=[]  NCopyOutDataTypeStr=Inherit: Inherit via back propagation  NCopyOutMin=[]  NCopyOutMax=[]  IntegratorContinuousStateAttributes=''  IntegratorStateMustResolveToSignalObject=off  IntegratorRTWStateStorageClass=Auto  FilterContinuousStateAttributes=''  FilterStateMustResolveToSignalObject=off  FilterRTWStateStorageClass=Auto  ParallelPVariant=InternalParameters  IdealPVariant=Disabled  IVariant=InternalParameters  DVariant=Disabled  IntegratorVariant=Continuous  SatVariant=Disabled  AWVariant=Passthrough  PCopyVariant=Disabled  TRVariant=Disabled  FdbkBlocksVariant=Forward  IdealPFdbkVariant=Disabled  SatFdbkVariant=Disabled  DerivativeFilterVariant=Disabled  NVariant=Disabled  NCopyVariant=Disabled_SignalSpec  FilterICVariant=Disabled  IntegratorICVariant=InternalICs  ExternalResetVariant=Disabled  TRSumVariant=Passthrough  SumFdbkVariant=Disabled  SumVariant=Sum_PI  TsampFilterVariant=InternalTs  TsampNgainVariant=Passthrough  TsampIntegralVariant=Disabled_SignalSpec  ExternalSaturationOutDataTypeStr=Inherit: Same as second input  DerivativeSourceVariant=Disabled  PreIntVariant=InternalPreInt
  Relational Operator3 : RelationalOperator  OutDataTypeStr=boolean  RndMeth=Simplest  InputSameDT=off
  Repeating Sequence1 : simulink/Sources/Repeating Sequence  rep_seq_t=[0 0.0001]  rep_seq_y=[0 1]
  Sum : Sum  Inputs=|+-
  Sum1 : Sum  Inputs=|+-
  PWM1 : Outport
  PWM2 : Outport  Port=2
  wires:
  PID Controller/1 -> Relational Operator3/1
  Repeating Sequence1/1 -> Relational Operator3/2
  Relational Operator3/1 -> Logical Operator3/1, PWM1/1
  Logical Operator3/1 -> PWM2/1
  IE1/1 -> Sum/2
  PID Controller1/1 -> Sum/1
  Sum/1 -> PID Controller/1
  Uderef/1 -> Sum1/1
  Udc/1 -> Sum1/2
  Sum1/1 -> PID Controller1/1

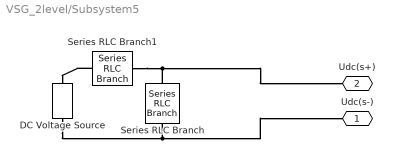
== system VSG_2level/Subsystem5 ==
  DC Voltage Source : spsDCVoltageSourceLib/DC Voltage Source  Amplitude=800  Measurements=None
  Series RLC Branch : spsSeriesRLCBranchLib/Series RLC Branch  LConnTagsString=__new0  RConnTagsString=__new0  BranchType=C  Resistance=1  Inductance=1e-3  SetiL0=off  InitialCurrent=0  Capacitance=1000e-6  Setx0=off  InitialVoltage=0  Measurements=None
  Series RLC Branch1 : spsSeriesRLCBranchLib/Series RLC Branch  LConnTagsString=__new0  RConnTagsString=__new0  BranchType=R  Resistance=0.000000000001  Inductance=1e-3  SetiL0=off  InitialCurrent=0  Capacitance=1000e-6  Setx0=off  InitialVoltage=0  Measurements=None
  Udc(s-) : PMIOPort  Side=Left
  Udc(s+) : PMIOPort  Port=2  Side=Left
  connections:
  Series RLC Branch1/LConn1 -- DC Voltage Source/RConn1
  Series RLC Branch/RConn1 -- Udc(s-)/RConn1 -- DC Voltage Source/LConn1
  Series RLC Branch1/RConn1 -- Udc(s+)/RConn1 -- Series RLC Branch/LConn1

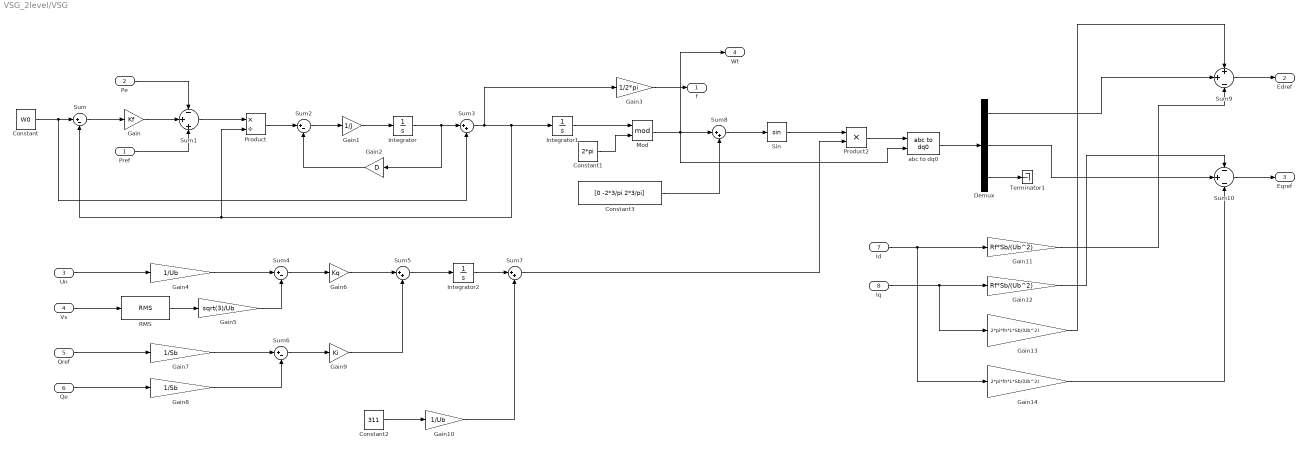
== system VSG_2level/VSG ==
  Pref : Inport
  Pe : Inport  Port=2
  Un : Inport  Port=3
  Vs : Inport  Port=4
  Qref : Inport  Port=5
  Qe : Inport  Port=6
  Id : Inport  Port=7
  Iq : Inport  Port=8
  Constant : Constant  Value=W0
  Constant1 : Constant  Value=2*pi
  Constant2 : Constant  Value=311
  Constant3 : Constant  Value=[0 -2*3/pi 2*3/pi]
  Demux : Demux  Outputs=3
  Gain : Gain  Gain=Kf
  Gain1 : Gain  Gain=1/J
  Gain10 : Gain  Gain=1/Ub
  Gain11 : Gain  Gain=Rf*Sb/(Ub^2)
  Gain12 : Gain  Gain=Rf*Sb/(Ub^2)
  Gain13 : Gain  Gain=2*pi*fn*L*Sb/(Ub^2)
  Gain14 : Gain  Gain=2*pi*fn*L*Sb/(Ub^2)
  Gain2 : Gain  Gain=D
  Gain3 : Gain  Gain=1/2*pi
  Gain4 : Gain  Gain=1/Ub
  Gain5 : Gain  Gain=sqrt(3)/Ub
  Gain6 : Gain  Gain=Kq
  Gain7 : Gain  Gain=1/Sb
  Gain8 : Gain  Gain=1/Sb
  Gain9 : Gain  Gain=Ki
  Integrator : Integrator  UpperSaturationLimit=100  LowerSaturationLimit=-100
  Integrator1 : Integrator
  Integrator2 : Integrator
  Mod : Math  Operator=mod
  Product : Product  Inputs=*/
  Product2 : Product
  RMS : dspstat3/RMS  run=off  directionMode=Each column  dimension=1  InputProcessing=Columns as channels (frame based)  reset_popup=None
  Sin : Trigonometry
  Sum{,2,4,6} (4 alike) : Sum  Inputs=|+-
  Sum1 : Sum  Inputs=-|+|+
  Sum10 : Sum  Inputs=-|+|-
  Sum{3,5,7..8} (4 alike) : Sum  Inputs=|++
  Sum9 : Sum  Inputs=+|+|-
  Terminator1 : Terminator
  abc to dq0 : spsabctodq0Lib/abc to dq0  Alignment=90 degrees behind phase A axis
  f : Outport
  Edref : Outport  Port=2
  Eqref : Outport  Port=3
  Wt : Outport  Port=4
  wires:
  Gain6/1 -> Sum5/1
  Gain2/1 -> Sum2/2
  Integrator2/1 -> Sum7/1
  Integrator1/1 -> Mod/1
  Id/1 -> Gain14/1, Gain11/1
  Demux/2 -> Sum10/2
  Un/1 -> Gain4/1
  Gain5/1 -> Sum4/2
  Sum5/1 -> Integrator2/1
  Gain13/1 -> Sum9/1
  Gain14/1 -> Sum10/3
  Gain9/1 -> Sum5/2
  Constant/1 -> Sum3/2, Sum/1
  Iq/1 -> Gain13/1, Gain12/1
  Gain/1 -> Sum1/2
  Sum6/1 -> Gain9/1
  Demux/1 -> Sum9/2
  abc to dq0/1 -> Demux/1
  Sum8/1 -> Sin/1
  Mod/1 -> Wt/1, abc to dq0/2, Sum8/1
  Qe/1 -> Gain8/1
  Demux/3 -> Terminator1/1
  Constant3/1 -> Sum8/2
  Sum4/1 -> Gain6/1
  Sum1/1 -> Product/1
  Product/1 -> Sum2/1
  Sum7/1 -> Product2/2
  Gain8/1 -> Sum6/2
  Gain10/1 -> Sum7/2
  Constant2/1 -> Gain10/1
  Gain12/1 -> Sum10/1
  Sum3/1 -> Gain3/1, Product/2, Sum/2, Integrator1/1
  Sum9/1 -> Edref/1
  Gain4/1 -> Sum4/1
  Qref/1 -> Gain7/1
  Gain7/1 -> Sum6/1
  Constant1/1 -> Mod/2
  Sin/1 -> Product2/1
  Gain11/1 -> Sum9/3
  RMS/1 -> Gain5/1
  Sum/1 -> Gain/1
  Gain3/1 -> f/1
  Sum2/1 -> Gain1/1
  Product2/1 -> abc to dq0/1
  Vs/1 -> RMS/1
  Sum10/1 -> Eqref/1
  Integrator/1 -> Gain2/1, Sum3/1
  Gain1/1 -> Integrator/1
  Pref/1 -> Sum1/3
  Pe/1 -> Sum1/1

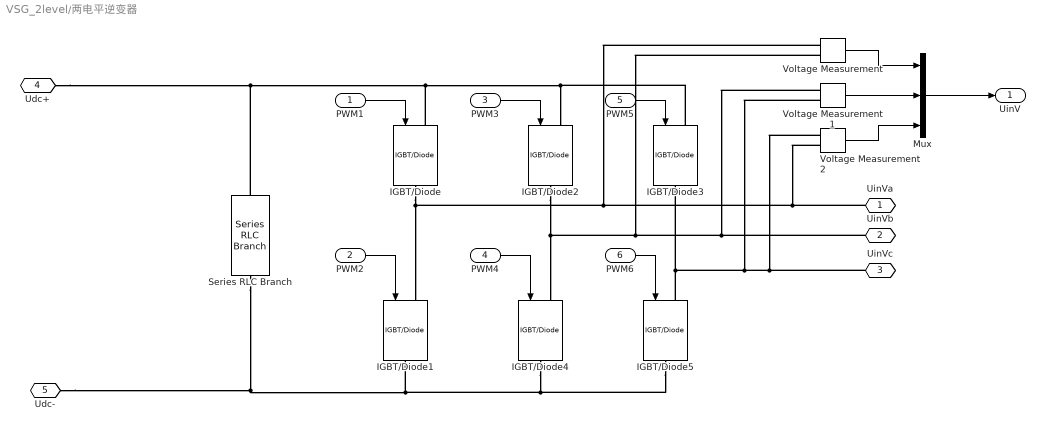
== system VSG_2level/两电平逆变器 ==
  PWM1 : Inport
  PWM2 : Inport  Port=2
  PWM3 : Inport  Port=3
  PWM4 : Inport  Port=4
  PWM5 : Inport  Port=5
  PWM6 : Inport  Port=6
  IGBT/Diode{,1..5} (6 alike) : spsIGBTDiodeLib/IGBT//Diode  Ron=1e-3  Rs=1e5  Cs=inf  Measurements=off
  Mux : Mux  Inputs=3
  Series RLC Branch : spsSeriesRLCBranchLib/Series RLC Branch  LConnTagsString=__new0  RConnTagsString=__new0  BranchType=RC  Resistance=1e-3  Inductance=1e-3  SetiL0=off  InitialCurrent=0  Capacitance=5000e-6  Setx0=on  InitialVoltage=800  Measurements=None
  Voltage Measurement : spsVoltageMeasurementLib/Voltage Measurement  PhasorSimulation=off  OutputType=Complex  PSBequivalent=0
  Voltage Measurement1 : spsVoltageMeasurementLib/Voltage Measurement  PhasorSimulation=off  OutputType=Complex  PSBequivalent=0
  Voltage Measurement2 : spsVoltageMeasurementLib/Voltage Measurement  PhasorSimulation=off  OutputType=Complex  PSBequivalent=0
  UinVa : PMIOPort  Side=Right
  UinVb : PMIOPort  Port=2  Side=Right
  UinVc : PMIOPort  Port=3  Side=Right
  Udc+ : PMIOPort  Port=4  Side=Left
  Udc- : PMIOPort  Port=5  Side=Left
  UinV : Outport
  wires:
  PWM6/1 -> IGBT/Diode5/1
  PWM3/1 -> IGBT/Diode2/1
  Voltage Measurement2/1 -> Mux/3
  PWM1/1 -> IGBT/Diode/1
  PWM5/1 -> IGBT/Diode3/1
  Mux/1 -> UinV/1
  PWM2/1 -> IGBT/Diode1/1
  Voltage Measurement1/1 -> Mux/2
  PWM4/1 -> IGBT/Diode4/1
  Voltage Measurement/1 -> Mux/1
  connections:
  IGBT/Diode/LConn1 -- Udc+/RConn1 -- Series RLC Branch/LConn1 -- IGBT/Diode3/LConn1 -- IGBT/Diode2/LConn1
  IGBT/Diode/RConn1 -- UinVa/RConn1 -- Voltage Measurement2/LConn2 -- Voltage Measurement/LConn1 -- IGBT/Diode1/LConn1
  IGBT/Diode4/RConn1 -- IGBT/Diode5/RConn1 -- Udc-/RConn1 -- Series RLC Branch/RConn1 -- IGBT/Diode1/RConn1
  IGBT/Diode5/LConn1 -- UinVc/RConn1 -- Voltage Measurement2/LConn1 -- Voltage Measurement1/LConn2 -- IGBT/Diode3/RConn1
  IGBT/Diode2/RConn1 -- UinVb/RConn1 -- Voltage Measurement1/LConn1 -- Voltage Measurement/LConn2 -- IGBT/Diode4/LConn1
